simulink model "C705_FLATEARTH_sim"  (R2016a)
settings: Solver=ode23tb  StartTime=0.0  StopTime=t_sim  FixedStep=Ts  RelTol=1e-2
values from neighbouring files (symbols this model uses):
  att0 = [deg2rad(phi0) deg2rad(theta0) deg2rad(psi0)]    [C705_FLATEARTH_init2.m]
  boost = 30000    [C705_CFD_parameter.m]
  C = [-0.00159261761698 -0.0785492193562 0 0 0 0 0 0 -0.0394443854537 -0.0139411758211 0 0 ... (48 elements, 1x48)]    [C705CFDv2.mat]
  C3to4 = [1 -1 1;1 1 1;-1 1 1;-1 -1 1]    [C705_CFD_parameter.m]    (also in C705_FLATEARTH_init2.m)
  C4to3 = (1/4)*[1 1 -1 -1;-1 1 1 -1;1 1 1 1]    [C705_CFD_parameter.m]    (also in C705_FLATEARTH_init2.m)
  d_transisi = 2e3    (= 2000)    [C705_FLATEARTH_init2.m]
  dela_max = deg2rad(10)    [C705_FLATEARTH_init2.m]
  dele_max = deg2rad(10)    [C705_FLATEARTH_init2.m]
  delr_max = deg2rad(10)    [C705_FLATEARTH_init2.m]
  dmdt = -m_fuel/tmax    (= -0.04)    [C705_CFD_parameter.m]
  f_camera = 0.1    [C705_FLATEARTH_init2.m]
  fmax = (10/180)*pi    (= 0.174532925199)    [C705_CFD_parameter.m]    (also in C705_FLATEARTH_init2.m = deg2rad(10))
  k0 = 1    [C705_FLATEARTH_init2.m]
  Khdot = -1    [C705_FLATEARTH_init2.m]
  Ki_ay = -0.0024    [C705_FLATEARTH_init2.m]
  Ki_az = 0.0085    [C705_FLATEARTH_init2.m]
  Ki_psi = 4.1865e-07    [C705_FLATEARTH_init2.m]
  Ki_theta = 2.1878e-7    (= 2.1878e-07)    [C705_FLATEARTH_init2.m]
  Kiphi = 2e-7    (= 2e-07)    [C705_FLATEARTH_init2.m]
  Kp = -1.3248    [C705_FLATEARTH_init2.m]
  Kp_ay = -0.0135    [C705_FLATEARTH_init2.m]
  Kp_az = 0.0119    [C705_FLATEARTH_init2.m]
  Kp_h = 0.45    [C705_FLATEARTH_init2.m]
  Kp_psi = 1.7937    [C705_FLATEARTH_init2.m]
  Kp_theta = 1.7024    [C705_FLATEARTH_init2.m]
  Kphi = 1.8594    [C705_FLATEARTH_init2.m]
  Kq = 3.8200    (= 3.82)    [C705_FLATEARTH_init2.m]
  Kq_theta = -3.1594    [C705_FLATEARTH_init2.m]
  Kr = -10.1447    [C705_FLATEARTH_init2.m]
  Kr_psi = 8.6031    [C705_FLATEARTH_init2.m]
  Lref = 3.675    [C705_CFD_parameter.m]
  m_init = m_full-m_boost    (= 286)    [C705_CFD_parameter.m]
  N = 3    [C705_FLATEARTH_init2.m]
  p0 = [0,0,-h0]    [C705_FLATEARTH_init2.m]
  p1 = [6000,100,-200]    [C705_FLATEARTH_init2.m]
  p2 = [12000,300,-200]    [C705_FLATEARTH_init2.m]
  p3 = [18000,700,-200]    [C705_FLATEARTH_init2.m]
  pt = [24000,1000,0]    [C705_FLATEARTH_init2.m]
  Sref = 0.1711917    [C705_CFD_parameter.m]
  t_activate_del_a = 3    [C705_FLATEARTH_init2.m]
  t_activate_del_e = 5    [C705_FLATEARTH_init2.m]
  t_activate_del_r = 5    [C705_FLATEARTH_init2.m]
  tboost = 3    [C705_FLATEARTH_init2.m]
  TH = 3    [C705_FLATEARTH_init2.m]
  thrust = 910    [C705_CFD_parameter.m]
  Ts_ap = 1/Fs_ap    (= 0.005)    [C705_FLATEARTH_init2.m]
  Ts_guid = 1/Fs_guid    (= 0.005)    [C705_FLATEARTH_init2.m]
  tswitch = 0    [C705_FLATEARTH_init2.m]
  vb0 = [1e-3 0 0]    [C705_FLATEARTH_init2.m]
  wb0 = [0 0 0]    [C705_FLATEARTH_init2.m]
undefined symbols (not defined in the file or in its folder): DiscIntNeverNeededParam, F, GIr, GPr, K1r, K2r, Kda, Ki_h, Ki_p, Kp_p, Light, MIL
libraries: simulink x11, aerolibasang x4, aerolibguid x3, aerolibwind2 x3, aerolibutil x2, aerolibanim x1, aerolibactuator x1, aerolibtransform2 x1, aerolibatmos2 x1, aerolibgravity2 x1, aerolibbdyn x1, aerolibnav x1
(part 1 of 2)
settings Model: Creator=tommypra97  LastModifiedBy=LABSSAJ204
settings DataIOCC: LimitDataPoints=on  SaveFormat=StructureWithTime  SignalLoggingSaveFormat=ModelDataLogs  SaveTime=off
settings DebuggingCC: FcnCallInpInsideContextMsg=EnableAllAsWarning
settings HardwareCC: ProdBitPerPointer=32  ProdLargestAtomicFloat=None  ProdWordSize=32  ProdHWDeviceType=Specified
settings ModelReferenceCC: PropagateSignalLabelsOutOfModel=off
settings GRTTargetCC: CombineOutputUpdateFcns=off  GRTInterface=on

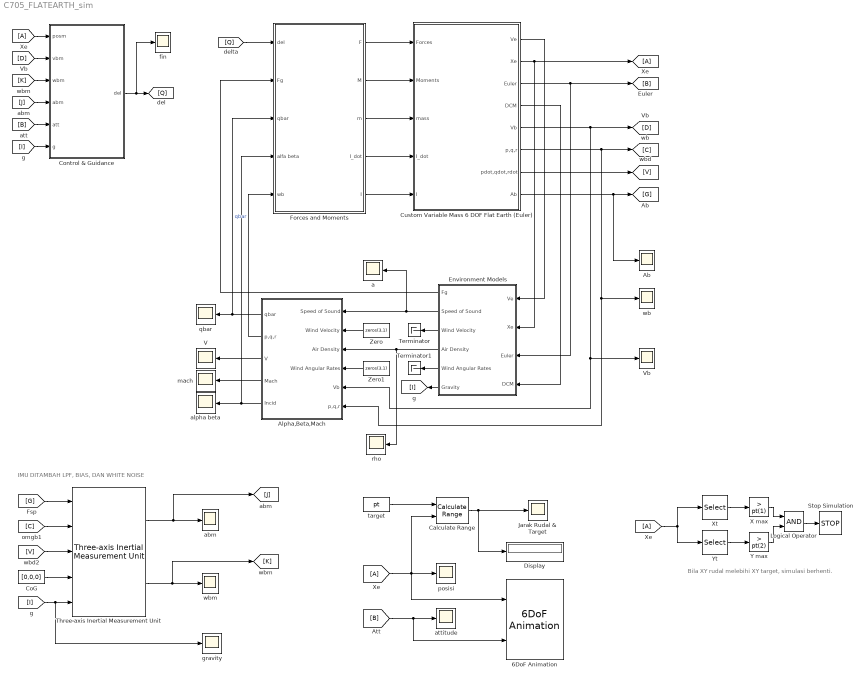
== system C705_FLATEARTH_sim ==
  note: Bila XY rudal melebihi XY target, simulasi berhenti.
  note: IMU DITAMBAH LPF, BIAS, DAN WHITE NOISE
  " Vb " : Scope
  " wb " : Scope
  6DoF Animation : aerolibanim/6DoF Animation  u1=[0 1 0 1 0 1]  u2=0.03  u3=7  u4=pt  u5=Fly alongside  u6=[-20 0 -7]  u7=20  u8=on
  "Ab " : Scope
  Alpha,Beta,Mach : Subsystem
  Calculate Range : aerolibguid/Calculate Range
  CoG : Constant  Value=[0,0,0]
  Control & Guidance : Subsystem
  Custom Variable Mass 6 DOF Flat Earth (Euler) : Subsystem
  Display : Display
  Environment Models : Subsystem
  Forces and Moments : Subsystem
  Jarak Rudal & Target : Scope
  Logical Operator : Logic  AllPortsSameDT=off  OutDataTypeStr=boolean
  Stop Simulation : Stop
  Terminator : Terminator
  Terminator1 : Terminator
  Three-axis Inertial Measurement Unit : aerolibnav/Three-axis Inertial Measurement Unit  units=Metric (MKS)  imu=[0 0 0]  dtype_a=on  w_a=wn_lpf  z_a=zeta_lpf  a_sf_cc=[1 0 0; 0 1 0; 0 0 1]  a_bias=acc_bias  a_sat="[-inf  -inf  -inf  inf inf inf]"  dtype_g=on  w_g=wn_lpf  z_g=zeta_lpf  g_sf_cc=[1 0 0; 0 1 0; 0 0 1]  g_bias=gyr_bias  g_sens=[0 0 0]  g_sat="[-inf  -inf  -inf  inf inf inf]"  i_rand=on  i_seeds=imu_noise_seed  i_pow=imu_noise_pwr  i_Ts=Ts_imu
  V : Scope
  X max : simulink/Logic and Bit Operations/Compare To Constant  relop=>  const=pt(1)  OutDataTypeStr=boolean  ZeroCross=off
  Xt : Selector  InputPortWidth=3  IndexOptions=Index vector (dialog)  Indices=1  OutputSizes=1
  Y max : simulink/Logic and Bit Operations/Compare To Constant  relop=>  const=pt(2)  OutDataTypeStr=boolean  ZeroCross=off
  Yt : Selector  InputPortWidth=3  IndexOptions=Index vector (dialog)  Indices=2  OutputSizes=1
  Zero : Constant  Value=zeros(3,1)
  Zero1 : Constant  Value=zeros(3,1)
  a : Scope
  "abm " : Scope
  alpha beta : Scope
  attitude : Scope
  "fin " : Scope
  gravity : Scope
  mach : Scope
  posisi : Scope
  qbar : Scope
  rho : Scope
  target : Constant  Value=pt
  "wbm " : Scope
  wires:
  Custom Variable Mass 6 DOF Flat Earth (Euler)/6(p,q,r) -> " wb "/1, Alpha,Beta,Mach/6(p,q,r), [C]
  Custom Variable Mass 6 DOF Flat Earth (Euler)/7(pdot,qdot,rdot) -> [V]
  Custom Variable Mass 6 DOF Flat Earth (Euler)/4(DCM) -> Environment Models/4(DCM)
  Custom Variable Mass 6 DOF Flat Earth (Euler)/3(Euler) -> [B], Environment Models/3(Euler)
  Environment Models/2(Speed of Sound) -> a/1, Alpha,Beta,Mach/1(Speed of Sound)
  Environment Models/4(Air Density) -> Alpha,Beta,Mach/3(Air Density), rho/1
  [A] -> Calculate Range/2, 6DoF Animation/1, posisi/1
  target/1 -> Calculate Range/1
  Alpha,Beta,Mach/4(Mach) -> mach/1
  Environment Models/1(Fg) -> Forces and Moments/2(Fg)
  Alpha,Beta,Mach/5(Incid) -> alpha beta/1, Forces and Moments/4(alfa beta)
  Environment Models/6(Gravity) -> [I]
  [G] -> Three-axis Inertial Measurement Unit/1
  [C] -> Three-axis Inertial Measurement Unit/2
  CoG/1 -> Three-axis Inertial Measurement Unit/4
  [I] -> Three-axis Inertial Measurement Unit/5, gravity/1
  [V] -> Three-axis Inertial Measurement Unit/3
  [A] -> Control & Guidance/1(posm)
  [D] -> Control & Guidance/2(vbm)
  [K] -> Control & Guidance/3(wbm)
  [J] -> Control & Guidance/4(abm)
  Custom Variable Mass 6 DOF Flat Earth (Euler)/8(Ab) -> "Ab "/1, [G]
  Alpha,Beta,Mach/1(qbar) -> qbar/1, Forces and Moments/3(qbar)  "qbar"
  Alpha,Beta,Mach/3(V) -> V/1
  Three-axis Inertial Measurement Unit/1 -> [J], "abm "/1
  Three-axis Inertial Measurement Unit/2 -> [K], "wbm "/1
  [B] -> Control & Guidance/5(att)
  Zero/1 -> Alpha,Beta,Mach/2(Wind Velocity)
  Zero1/1 -> Alpha,Beta,Mach/4(Wind Angular Rates)
  Environment Models/3(Wind Velocity) -> Terminator/1
  Environment Models/5(Wind Angular Rates) -> Terminator1/1
  [Q] -> Forces and Moments/1(del)
  Calculate Range/1 -> Display/1, Jarak Rudal & Target/1
  [I] -> Control & Guidance/6(g)
  Control & Guidance/1(del) -> "fin "/1, [Q]
  Alpha,Beta,Mach/2("p,q,r ") -> Forces and Moments/5(wb)
  Custom Variable Mass 6 DOF Flat Earth (Euler)/5(Vb) -> Alpha,Beta,Mach/5(Vb), " Vb "/1, [D]
  Forces and Moments/1(F) -> Custom Variable Mass 6 DOF Flat Earth (Euler)/1(Forces)
  Forces and Moments/2(M) -> Custom Variable Mass 6 DOF Flat Earth (Euler)/2(Moments)
  [B] -> attitude/1, 6DoF Animation/2
  Y max/1 -> Logical Operator/2
  X max/1 -> Logical Operator/1
  Logical Operator/1 -> Stop Simulation/1
  Xt/1 -> X max/1
  Yt/1 -> Y max/1
  Custom Variable Mass 6 DOF Flat Earth (Euler)/2(Xe) -> [A], Environment Models/2(Xe)
  Forces and Moments/5(I) -> Custom Variable Mass 6 DOF Flat Earth (Euler)/5(I)
  Forces and Moments/3(m) -> Custom Variable Mass 6 DOF Flat Earth (Euler)/3(mass)
  Forces and Moments/4(I_dot) -> Custom Variable Mass 6 DOF Flat Earth (Euler)/4(I_dot)
  Custom Variable Mass 6 DOF Flat Earth (Euler)/1(Ve) -> Environment Models/1(Ve)
  [A] -> Yt/1, Xt/1

== system C705_FLATEARTH_sim/Alpha,Beta,Mach ==
  Speed of Sound : Inport
  Wind Velocity : Inport  Port=2  PortDimensions=3
  Air Density : Inport  Port=3
  Wind Angular Rates : Inport  Port=4  PortDimensions=3
  Vb : Inport  Port=5  PortDimensions=3
  p,q,r : Inport  Port=6  PortDimensions=3
  Dynamic Pressure : aerolibasang/Dynamic Pressure
  "Incidence, Sideslip & Airspeed" : aerolibasang/Incidence, Sideslip, & Airspeed
  Mach Number : aerolibasang/Mach Number
  Mux : Mux  Inputs=2
  Sum : Sum  Inputs=|+-  SaturateOnIntegerOverflow=on  InputSameDT=on  OutDataTypeStr=Inherit: Same as first input
  Sum1 : Sum  Inputs=|++  SaturateOnIntegerOverflow=on  InputSameDT=on  OutDataTypeStr=Inherit: Same as first input
  qbar : Outport  InitialOutput=0
  "p,q,r " : Outport  Port=2
  V : Outport  Port=3
  Mach : Outport  Port=4
  Incid : Outport  Port=5
  wires:
  "Incidence, Sideslip & Airspeed"/3 -> V/1
  Dynamic Pressure/1 -> qbar/1
  Air Density/1 -> Dynamic Pressure/2
  Mach Number/1 -> Mach/1
  Sum/1 -> Dynamic Pressure/1, Mach Number/1, "Incidence, Sideslip & Airspeed"/1
  Vb/1 -> Sum/1
  Speed of Sound/1 -> Mach Number/2
  Wind Velocity/1 -> Sum/2
  "Incidence, Sideslip & Airspeed"/2 -> Mux/2  "Beta"
  Mux/1 -> Incid/1
  "Incidence, Sideslip & Airspeed"/1 -> Mux/1  "Alpha"
  p,q,r/1 -> Sum1/1
  Wind Angular Rates/1 -> Sum1/2
  Sum1/1 -> "p,q,r "/1

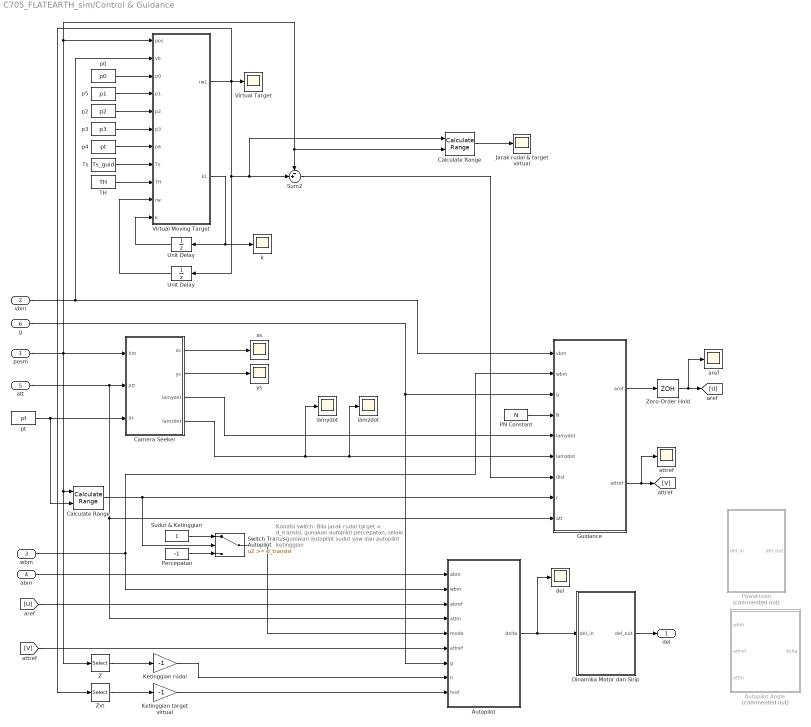
== system C705_FLATEARTH_sim/Control & Guidance ==
  note: Kondisi switch:
      | Bila jarak rudal-target < d_transisi,
      | gunakan autopilot percepatan,
      | selain itu, gunakan autopilot sudut yaw dan
      | autopilot ketinggian
  posm : Inport
  vbm : Inport  Port=2
  wbm : Inport  Port=3
  abm : Inport  Port=4
  att : Inport  Port=5
  g : Inport  Port=6
  Autopilot : Subsystem
  Autopilot Angle : Subsystem  Commented=on
  Calculate Range : aerolibguid/Calculate Range
  "Calculate Range " : aerolibguid/Calculate Range
  Camera Seeker : Subsystem
  Dinamika Motor dan Sirip : Subsystem
  Guidance : MATLAB Function  TreatAsAtomicUnit=on
  Jarak rudal & target virtual : Scope
  Ketinggian rudal : Gain  Gain=-1
  Ketinggian target virtual : Gain  Gain=-1
  PN Constant : Constant  Value=N
  Percepatan : Constant  Value=-1
  Pewaktuan : Subsystem  Commented=on
  Sudut & Ketinggian : Constant
  Sum2 : Sum  Inputs=-+|
  Switch Transisi Autopilot : Switch  Threshold=d_transisi
  TH : Constant  Value=TH
  Ts : Constant  Value=Ts_guid
  Unit Delay : UnitDelay  InitialCondition=k0  SampleTime=Ts_guid
  "Unit Delay " : UnitDelay  InitialCondition=p1  SampleTime=Ts_guid
  Virtual Moving Target : MATLAB Function  TreatAsAtomicUnit=on
  Virtual Target : Scope
  Z : Selector  InputPortWidth=3  IndexOptions=Index vector (dialog)  Indices=[3]  OutputSizes=1
  Zero-Order Hold : ZeroOrderHold  SampleTime=Ts_guid
  Zvt : Selector  InputPortWidth=3  IndexOptions=Index vector (dialog)  Indices=[3]  OutputSizes=1
  "aref " : Scope
  "attref " : Scope
  "del " : Scope
  k : Scope
  lamydot : Scope
  lamzdot : Scope
  p0 : Constant  Value=p0  VectorParams1D=off
  p2 : Constant  Value=p2
  p3 : Constant  Value=p3
  p4 : Constant  Value=pt
  p5 : Constant  Value=p1
  pt : Constant  Value=pt
  xs : Scope
  ys : Scope
  del : Outport
  wires:
  abm/1 -> Autopilot/1(abm)
  wbm/1 -> Autopilot/2(wbm), Guidance/2(wbm)
  g/1 -> Guidance/3(g), Autopilot/7(g)
  PN Constant/1 -> Guidance/4(N)
  Camera Seeker/1(xs) -> xs/1
  Camera Seeker/2(ys) -> ys/1
  Camera Seeker/3(lamydot) -> Guidance/5(lamydot)
  Camera Seeker/4(lamzdot) -> lamydot/1, lamzdot/1, Guidance/6(lamzdot)
  Zero-Order Hold/1 -> "aref "/1, [U]
  [U] -> Autopilot/3(abref)
  Guidance/1(aref) -> Zero-Order Hold/1
  p5/1 -> Virtual Moving Target/4(p1)
  p2/1 -> Virtual Moving Target/5(p2)
  p3/1 -> Virtual Moving Target/6(p3)
  p4/1 -> Virtual Moving Target/7(p4)
  vbm/1 -> Guidance/1(vbm), Virtual Moving Target/2(vb)
  Ts/1 -> Virtual Moving Target/8(Ts)
  "Unit Delay "/1 -> Virtual Moving Target/10(rw)
  Virtual Moving Target/2(k1) -> k/1, Unit Delay/1
  TH/1 -> Virtual Moving Target/9(TH)
  Unit Delay/1 -> Virtual Moving Target/11(k)
  p0/1 -> Virtual Moving Target/3(p0)
  Sum2/1 -> Guidance/7(dist)
  Guidance/2(attref) -> [V], "attref "/1
  posm/1 -> Calculate Range/1, Z/1, "Calculate Range "/2, Sum2/1, Virtual Moving Target/1(pos), Camera Seeker/1(Xm)
  pt/1 -> Calculate Range/2, Camera Seeker/3(Xt)
  "Calculate Range "/1 -> Jarak rudal & target virtual/1
  Calculate Range/1 -> Guidance/8(r), Switch Transisi Autopilot/2
  Autopilot/1(delta) -> "del "/1, Dinamika Motor dan Sirip/1(del_in)
  Dinamika Motor dan Sirip/1(del_out) -> del/1
  att/1 -> Guidance/9(att), Autopilot/4(attm), Camera Seeker/2(Att)
  Switch Transisi Autopilot/1 -> Autopilot/5(mode)
  Percepatan/1 -> Switch Transisi Autopilot/3
  Sudut & Ketinggian/1 -> Switch Transisi Autopilot/1
  [V] -> Autopilot/6(attref)
  Z/1 -> Ketinggian rudal/1
  Ketinggian rudal/1 -> Autopilot/8(h)
  Zvt/1 -> Ketinggian target virtual/1
  Ketinggian target virtual/1 -> Autopilot/9(href)
  Virtual Moving Target/1(rw1) -> Zvt/1, "Calculate Range "/1, Sum2/2, "Unit Delay "/1, Virtual Target/1

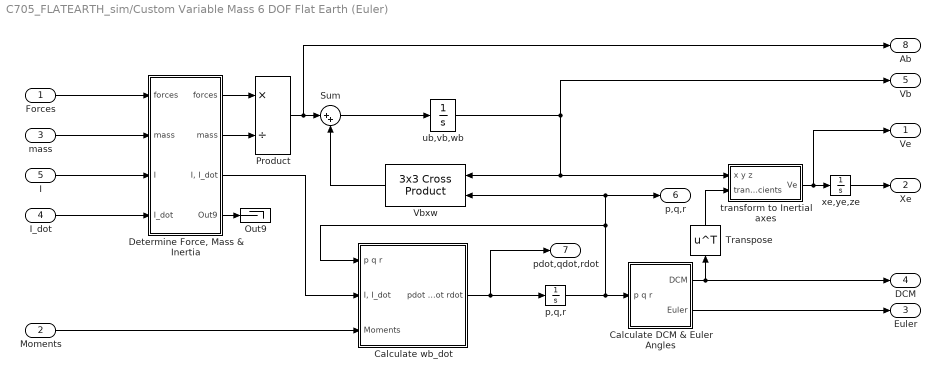
== system C705_FLATEARTH_sim/Custom Variable Mass 6 DOF Flat Earth (Euler) ==
  Forces : Inport  PortDimensions=3
  Moments : Inport  Port=2  PortDimensions=3
  mass : Inport  Port=3
  I_dot : Inport  Port=4  PortDimensions=[3 3]
  I : Inport  Port=5  PortDimensions=[3 3]
  Calculate DCM & Euler Angles : Subsystem
  "Calculate wb_dot " : Subsystem
  "Determine Force, Mass & Inertia " : Subsystem
  Out9 : Terminator
  Product : Product  Inputs=*/  SaturateOnIntegerOverflow=on  OutDataTypeStr=Inherit: Same as first input
  Sum : Sum  Inputs=|++  SaturateOnIntegerOverflow=on
  Transpose : Math  Operator=transpose  SaturateOnIntegerOverflow=on
  Vbxw : aerolibutil/3x3 Cross Product
  "p,q,r " : Integrator  InitialCondition=wb0
  transform to Inertial axes : Subsystem
  ub,vb,wb : Integrator  InitialCondition=vb0
  xe,ye,ze : Integrator  InitialCondition=p0
  Ve : Outport
  Xe : Outport  Port=2
  Euler : Outport  Port=3
  DCM : Outport  Port=4
  Vb : Outport  Port=5
  p,q,r : Outport  Port=6
  pdot,qdot,rdot : Outport  Port=7
  Ab : Outport  Port=8
  wires:
  Sum/1 -> ub,vb,wb/1
  "Determine Force, Mass & Inertia "/1("forces ") -> Product/1
  I_dot/1 -> "Determine Force, Mass & Inertia "/4(I_dot)
  "Calculate wb_dot "/1(pdot qdot rdot) -> pdot,qdot,rdot/1, "p,q,r "/1
  "Determine Force, Mass & Inertia "/4(Out9) -> Out9/1
  "Determine Force, Mass & Inertia "/2(mass) -> Product/2
  mass/1 -> "Determine Force, Mass & Inertia "/2("mass ")
  Transpose/1 -> transform to Inertial axes/2(transform coefficients)
  Calculate DCM & Euler Angles/1(DCM) -> DCM/1, Transpose/1
  ub,vb,wb/1 -> Vb/1, transform to Inertial axes/1(x y z), Vbxw/1
  transform to Inertial axes/1(Ve) -> Ve/1, xe,ye,ze/1
  Product/1 -> Ab/1, Sum/1
  Forces/1 -> "Determine Force, Mass & Inertia "/1(forces)
  I/1 -> "Determine Force, Mass & Inertia "/3(I)
  Moments/1 -> "Calculate wb_dot "/3(Moments)
  "p,q,r "/1 -> Calculate DCM & Euler Angles/1("p q r "), "Calculate wb_dot "/1(p q r), p,q,r/1, Vbxw/2
  Calculate DCM & Euler Angles/2(Euler) -> Euler/1
  Vbxw/1 -> Sum/2
  xe,ye,ze/1 -> Xe/1
  "Determine Force, Mass & Inertia "/3("I, I_dot ") -> "Calculate wb_dot "/2("I, I_dot")

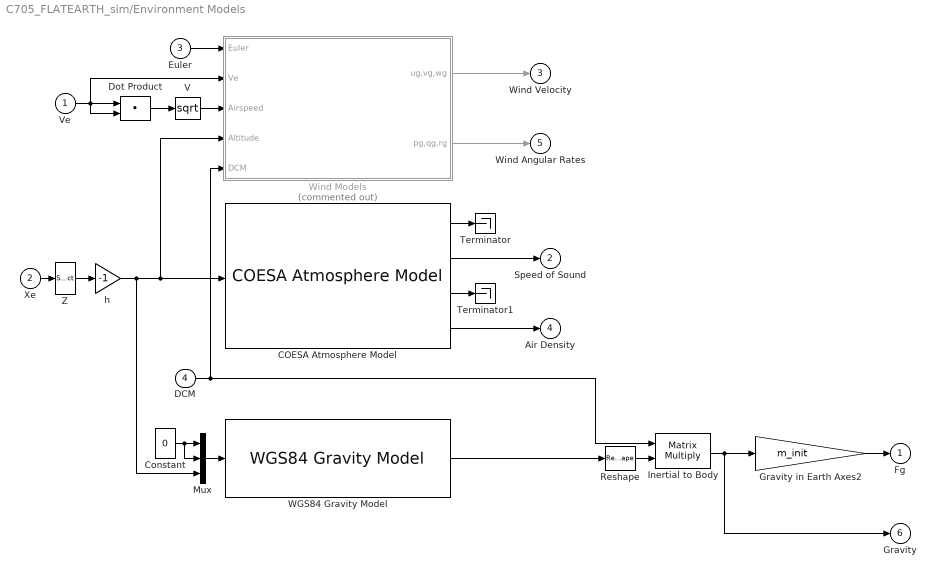
== system C705_FLATEARTH_sim/Environment Models ==
  Ve : Inport
  Xe : Inport  Port=2  PortDimensions=3
  Euler : Inport  Port=3
  DCM : Inport  Port=4
  COESA Atmosphere Model : aerolibatmos2/COESA Atmosphere Model  units=Metric (MKS)  spec=1976 COESA-extended U.S. Standard Atmosphere  model=Profile  profile_var=High temperature  profile_percent=10%  profile_alt=5 km (16404 ft)  envelope_var=High temperature  envelope_percent=1%  action=None
  Constant : Constant  Value=0
  Dot Product : DotProduct  SaturateOnIntegerOverflow=on  OutDataTypeStr=Inherit: Inherit via internal rule
  Gravity in Earth Axes2 : Gain  Gain=m_init  SaturateOnIntegerOverflow=on  OutDataTypeStr=Inherit: Same as input  ParamDataTypeStr=Inherit: Same as input
  Inertial to Body : Product  Multiplication=Matrix(*)  SaturateOnIntegerOverflow=on  InputSameDT=on  OutDataTypeStr=Inherit: Same as first input
  Mux : Mux  Inputs=3
  Reshape : Reshape
  Terminator : Terminator
  Terminator1 : Terminator
  V : Math  Operator=sqrt  SaturateOnIntegerOverflow=on
  "WGS84 Gravity Model " : aerolibgravity2/WGS84 Gravity Model   model=WGS84 Taylor Series  units=Metric (MKS)  no_atmos=on  precessing=on  jd_loc=off  month=October  day=10  year=2004  no_centrifugal=on  action=None
  Wind Models : Subsystem  Commented=on
  Z : Selector  InputPortWidth=3  IndexOptions=Index vector (dialog)  Indices=[3]  OutputSizes=1
  h : Gain  Gain=-1  SaturateOnIntegerOverflow=on  OutDataTypeStr=Inherit: Same as input  ParamDataTypeStr=Inherit: Same as input
  Fg : Outport  InitialOutput=0
  Speed of Sound : Outport  Port=2  InitialOutput=0
  Wind Velocity : Outport  Port=3  InitialOutput=0
  Air Density : Outport  Port=4  InitialOutput=0
  Wind Angular Rates : Outport  Port=5  InitialOutput=0
  Gravity : Outport  Port=6  InitialOutput=0
  wires:
  Reshape/1 -> Inertial to Body/2
  Euler/1 -> Wind Models/1(Euler)
  Ve/1 -> Wind Models/2(Ve), Dot Product/1, Dot Product/2
  Wind Models/1(ug,vg,wg) -> Wind Velocity/1
  Wind Models/2(pg,qg,rg) -> Wind Angular Rates/1
  Dot Product/1 -> V/1
  Z/1 -> h/1
  COESA Atmosphere Model/4 -> Air Density/1
  COESA Atmosphere Model/2 -> Speed of Sound/1
  COESA Atmosphere Model/3 -> Terminator1/1
  COESA Atmosphere Model/1 -> Terminator/1
  DCM/1 -> Wind Models/5(DCM), Inertial to Body/1
  V/1 -> Wind Models/3(Airspeed)
  "WGS84 Gravity Model "/1 -> Reshape/1
  Xe/1 -> Z/1
  Inertial to Body/1 -> Gravity/1, Gravity in Earth Axes2/1
  Gravity in Earth Axes2/1 -> Fg/1
  Mux/1 -> "WGS84 Gravity Model "/1
  Constant/1 -> Mux/2, Mux/1
  h/1 -> Mux/3, COESA Atmosphere Model/1, Wind Models/4(Altitude)

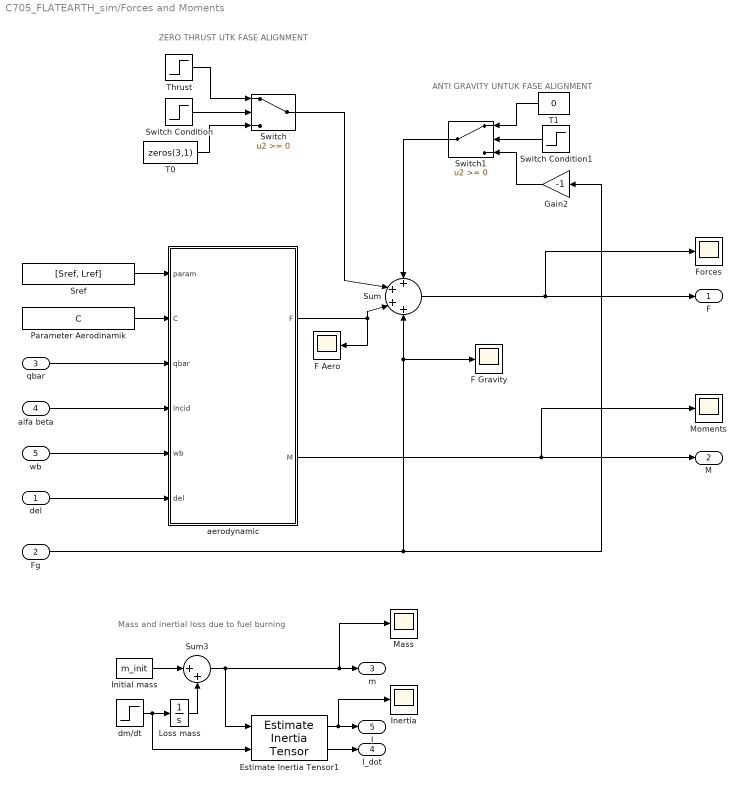
== system C705_FLATEARTH_sim/Forces and Moments ==
  note: ZERO THRUST UTK FASE ALIGNMENT
  note: ANTI GRAVITY UNTUK FASE ALIGNMENT
  note: Mass and inertial loss due to fuel burning
  del : Inport
  Fg : Inport  Port=2
  qbar : Inport  Port=3
  alfa beta : Inport  Port=4
  wb : Inport  Port=5
  " dm/dt " : Step  Time=tboost  Before=dmdt  After=0  SampleTime=0
  Estimate Inertia Tensor1 : aerolibbdyn/Estimate Inertia Tensor  fmass=m_init  emass=m_end  fI=I_init  eI=I_end
  F Aero : Scope
  F Gravity : Scope
  Forces : Scope
  Gain2 : Gain  Gain=-1
  "Inertia " : Scope
  Initial mass : Constant  Value=m_init
  Loss mass : Integrator
  Mass : Scope
  Moments : Scope
  Parameter Aerodinamik : Constant  Value=C  SampleTime=Ts_guid
  Sref : Constant  Value=[Sref, Lref]  SampleTime=Ts_guid
  Sum : Sum  Inputs=+|+|+|+  SaturateOnIntegerOverflow=on  InputSameDT=on  OutDataTypeStr=Inherit: Same as first input
  Sum3 : Sum  Inputs=|++  SaturateOnIntegerOverflow=on  InputSameDT=on  OutDataTypeStr=Inherit: Same as first input
  Switch : Switch
  Switch Condition : Step  Time=tswitch  Before=-1  SampleTime=0
  Switch Condition1 : Step  Time=tswitch  Before=-1  SampleTime=0
  Switch1 : Switch
  T0 : Constant  Value=zeros(3,1)  SampleTime=Ts_guid
  T1 : Constant  Value=0  SampleTime=Ts_guid
  Thrust : Step  Time=tswitch+tboost  Before=[boost 0 0]  After=[thrust 0 0]  SampleTime=0
  aerodynamic : MATLAB Function  TreatAsAtomicUnit=on
  F : Outport
  M : Outport  Port=2
  m : Outport  Port=3
  I_dot : Outport  Port=4
  I : Outport  Port=5
  wires:
  alfa beta/1 -> aerodynamic/4(incid)
  aerodynamic/1(F) -> Sum/3, F Aero/1
  qbar/1 -> aerodynamic/3(qbar)
  Sum/1 -> F/1, Forces/1
  Sref/1 -> aerodynamic/1(param)
  Parameter Aerodinamik/1 -> aerodynamic/2(C)
  aerodynamic/2(M) -> Moments/1, M/1
  del/1 -> aerodynamic/6(del)
  Switch Condition/1 -> Switch/2
  T0/1 -> Switch/3
  Thrust/1 -> Switch/1
  Switch Condition1/1 -> Switch1/2
  Gain2/1 -> Switch1/3
  T1/1 -> Switch1/1
  Switch1/1 -> Sum/1
  Switch/1 -> Sum/2
  wb/1 -> aerodynamic/5(wb)
  Fg/1 -> Sum/4, F Gravity/1, Gain2/1
  Estimate Inertia Tensor1/2 -> I_dot/1
  Estimate Inertia Tensor1/1 -> "Inertia "/1, I/1
  Initial mass/1 -> Sum3/1
  " dm/dt "/1 -> Estimate Inertia Tensor1/2, Loss mass/1
  Loss mass/1 -> Sum3/2
  Sum3/1 -> Estimate Inertia Tensor1/1, Mass/1, m/1

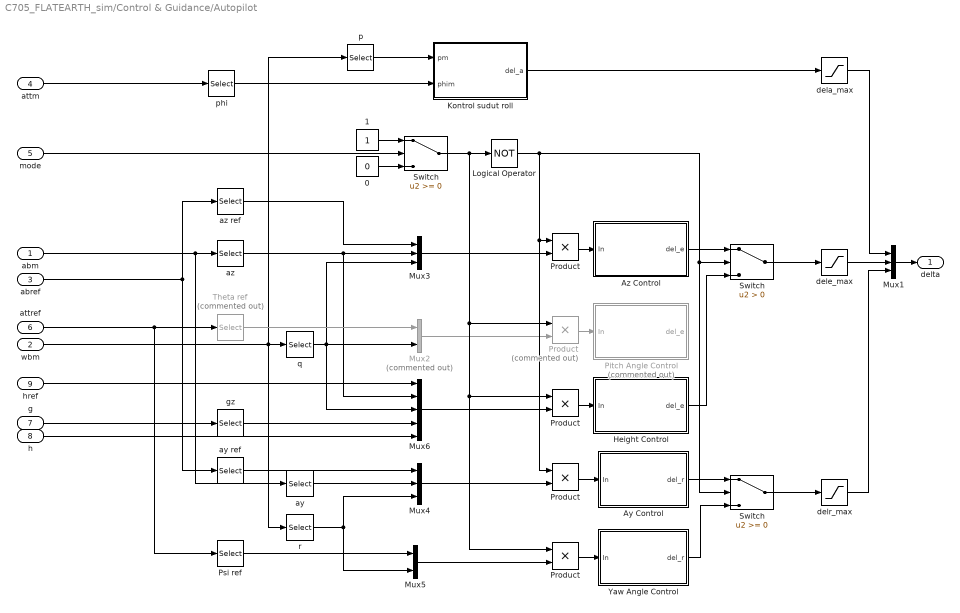
== system C705_FLATEARTH_sim/Control & Guidance/Autopilot ==
  abm : Inport
  wbm : Inport  Port=2
  abref : Inport  Port=3
  attm : Inport  Port=4
  mode : Inport  Port=5
  attref : Inport  Port=6
  g : Inport  Port=7
  h : Inport  Port=8
  href : Inport  Port=9
  " Product " : Product
  0 : Constant  Value=0
  1 : Constant
  Ay Control : Subsystem
  Az Control : Subsystem
  Height Control : Subsystem
  Kontrol sudut roll : Subsystem
  Logical Operator : Logic  Operator=NOT  AllPortsSameDT=off  OutDataTypeStr=boolean
  Mux1 : Mux  Inputs=3
  Mux2 : Mux  Commented=on  Inputs=2
  Mux3 : Mux  Inputs=3
  Mux4 : Mux  Inputs=3
  Mux5 : Mux  Inputs=2
  Mux6 : Mux  Inputs=5
  Pitch Angle Control : Subsystem  Commented=on
  Product : Product
  "Product " : Product  Commented=on
  "Product  " : Product
  "Product   " : Product
  Psi ref : Selector  InputPortWidth=3  IndexOptions=Index vector (dialog)  Indices=[3]  OutputSizes=1
  Switch : Switch
  "Switch " : Switch  Criteria=u2 > Threshold
  "Switch  " : Switch
  Theta ref : Selector  Commented=on  InputPortWidth=3  IndexOptions=Index vector (dialog)  Indices=2  OutputSizes=1
  Yaw Angle Control : Subsystem
  ay : Selector  InputPortWidth=3  IndexOptions=Index vector (dialog)  Indices=[2]  OutputSizes=1
  ay ref : Selector  InputPortWidth=3  IndexOptions=Index vector (dialog)  Indices=[2]  OutputSizes=1
  "az " : Selector  InputPortWidth=3  IndexOptions=Index vector (dialog)  Indices=[3]  OutputSizes=1
  az ref : Selector  InputPortWidth=3  IndexOptions=Index vector (dialog)  Indices=[3]  OutputSizes=1
  dela_max : Saturate  UpperLimit=dela_max  LowerLimit=-dela_max
  dele_max : Saturate  UpperLimit=dele_max  LowerLimit=-dele_max
  delr_max : Saturate  UpperLimit=delr_max  LowerLimit=-delr_max
  gz : Selector  InputPortWidth=3  IndexOptions=Index vector (dialog)  Indices=[3]  OutputSizes=1
  p : Selector  InputPortWidth=3  IndexOptions=Index vector (dialog)  Indices=[1]  OutputSizes=1
  phi : Selector  InputPortWidth=3  IndexOptions=Index vector (dialog)  Indices=[1]  OutputSizes=1
  q : Selector  InputPortWidth=3  IndexOptions=Index vector (dialog)  Indices=[2]  OutputSizes=1
  r : Selector  InputPortWidth=3  IndexOptions=Index vector (dialog)  Indices=[3]  OutputSizes=1
  delta : Outport
  wires:
  abref/1 -> az ref/1, ay ref/1
  wbm/1 -> q/1, p/1, r/1
  abm/1 -> "az "/1, ay/1
  p/1 -> Kontrol sudut roll/1(pm)
  Kontrol sudut roll/1(del_a) -> dela_max/1
  r/1 -> Mux5/2, Mux4/3
  az ref/1 -> Mux3/1
  attm/1 -> phi/1
  phi/1 -> Kontrol sudut roll/2(phim)
  dele_max/1 -> Mux1/2
  dela_max/1 -> Mux1/1
  delr_max/1 -> Mux1/3
  Mux1/1 -> delta/1
  q/1 -> Mux6/3, Mux3/3, Mux2/2
  mode/1 -> Switch/2
  0/1 -> Switch/3
  "az "/1 -> Mux6/2, Mux3/2
  Mux3/1 -> Product/2
  1/1 -> Switch/1
  Theta ref/1 -> Mux2/1
  Mux2/1 -> "Product "/2
  Switch/1 -> " Product "/1, "Product   "/1, "Product "/1, Logical Operator/1
  "Product "/1 -> Pitch Angle Control/1(In)
  Logical Operator/1 -> "Switch "/2, "Switch  "/2, "Product  "/1, Product/1
  Product/1 -> Az Control/1(In)
  ay ref/1 -> Mux4/1
  ay/1 -> Mux4/2
  Psi ref/1 -> Mux5/1
  Mux4/1 -> "Product  "/2
  Mux5/1 -> "Product   "/2
  "Product   "/1 -> Yaw Angle Control/1(In)
  "Product  "/1 -> Ay Control/1(In)
  Az Control/1(del_e) -> "Switch "/1
  Height Control/1(del_e) -> "Switch "/3
  "Switch "/1 -> dele_max/1
  Ay Control/1(del_r) -> "Switch  "/1
  Yaw Angle Control/1(del_r) -> "Switch  "/3
  "Switch  "/1 -> delr_max/1
  attref/1 -> Psi ref/1, Theta ref/1
  g/1 -> gz/1
  gz/1 -> Mux6/4
  " Product "/1 -> Height Control/1(In)
  Mux6/1 -> " Product "/2
  href/1 -> Mux6/1
  h/1 -> Mux6/5

== system C705_FLATEARTH_sim/Control & Guidance/Autopilot Angle ==
  wbm : Inport
  attref : Inport  Port=2
  attm : Inport  Port=3
  "Incidence, Sideslip & Airspeed" : aerolibasang/Incidence, Sideslip, & Airspeed  Commented=on
  Mux1 : Mux  Inputs=3
  Pitch Angle Control : Subsystem
  Psi ref : Selector  InputPortWidth=3  IndexOptions=Index vector (dialog)  Indices=[3]  OutputSizes=1
  Theta ref : Selector  InputPortWidth=3  IndexOptions=Index vector (dialog)  Indices=2  OutputSizes=1
  Yaw Angle Control : Subsystem
  p : Selector  InputPortWidth=3  IndexOptions=Index vector (dialog)  Indices=[1]  OutputSizes=1
  phi : Selector  InputPortWidth=3  IndexOptions=Index vector (dialog)  Indices=[1]  OutputSizes=1
  q : Selector  InputPortWidth=3  IndexOptions=Index vector (dialog)  Indices=[2]  OutputSizes=1
  r : Selector  InputPortWidth=3  IndexOptions=Index vector (dialog)  Indices=[3]  OutputSizes=1
  roll control : Subsystem
  delta : Outport
  wires:
  attref/1 -> Theta ref/1, Psi ref/1
  wbm/1 -> q/1, p/1, r/1
  p/1 -> roll control/1(pm)
  r/1 -> Yaw Angle Control/2("r ")
  q/1 -> Pitch Angle Control/2(q)
  Theta ref/1 -> Pitch Angle Control/1(Theta ref)
  Psi ref/1 -> Yaw Angle Control/1(Psi ref)
  Pitch Angle Control/1(del_e) -> Mux1/2
  roll control/1(del_a) -> Mux1/1
  Yaw Angle Control/1(del_r) -> Mux1/3
  Mux1/1 -> delta/1
  attm/1 -> phi/1
  phi/1 -> roll control/2(phim)

== system C705_FLATEARTH_sim/Control & Guidance/Camera Seeker ==
  Xm : Inport
  Att : Inport  Port=2
  Xt : Inport  Port=3
  Derivative : Derivative
  "Derivative " : Derivative
  Screen Camera : MATLAB Function  TreatAsAtomicUnit=on
  camera focus : Constant  Value=f_camera
  lamy : Scope
  lamz : Scope
  limit : Saturate  UpperLimit=pi  LowerLimit=-pi  LinearizeAsGain=off  ZeroCross=off
  limit1 : Saturate  UpperLimit=pi  LowerLimit=-pi  LinearizeAsGain=off  ZeroCross=off
  xs : Outport
  ys : Outport  Port=2
  lamydot : Outport  Port=3
  lamzdot : Outport  Port=4
  wires:
  Screen Camera/2(ys) -> ys/1
  Screen Camera/1(xs) -> xs/1
  Att/1 -> Screen Camera/2(att)
  Xm/1 -> Screen Camera/1(xm)
  Xt/1 -> Screen Camera/3(xt)
  camera focus/1 -> Screen Camera/4(f)
  Screen Camera/3(lamy) -> lamy/1, Derivative/1
  Screen Camera/4(lamz) -> lamz/1, "Derivative "/1
  "Derivative "/1 -> limit1/1
  Derivative/1 -> limit/1
  limit1/1 -> lamzdot/1
  limit/1 -> lamydot/1

== system C705_FLATEARTH_sim/Control & Guidance/Dinamika Motor dan Sirip ==
  del_in : Inport
  Act2Aero : Gain  Gain=C4to3  Multiplication=Matrix(K*u)  SaturateOnIntegerOverflow=on  OutDataTypeStr=Inherit: Same as input  ParamDataTypeStr=Inherit: Same as input
  Aero2Act : Gain  Gain=C3to4  Multiplication=Matrix(K*u)  SaturateOnIntegerOverflow=on  OutDataTypeStr=Inherit: Same as input  ParamDataTypeStr=Inherit: Same as input
  Nonlinear Second-Order Actuator : aerolibactuator/Nonlinear Second-Order Actuator  wn_fin=wn_act  z_fin=zeta_act  fin_max=[fmax fmax fmax fmax]  fin_min=-[fmax fmax fmax fmax]  fin_maxrate=inf  fin_act_0=0  fin_act_vel=0
  Scope1 : Scope
  Scope3 : Scope
  del_out : Outport
  wires:
  Act2Aero/1 -> del_out/1
  del_in/1 -> Aero2Act/1
  Aero2Act/1 -> Nonlinear Second-Order Actuator/1, Scope1/1
  Nonlinear Second-Order Actuator/1 -> Scope3/1, Act2Aero/1

== system C705_FLATEARTH_sim/Control & Guidance/Pewaktuan ==
  del_in : Inport
  Demux1 : Demux  Outputs=3
  Mux3 : Mux  Inputs=3
  Switch Condition : Step  Time=t_activate_del_a  Before=-1  SampleTime=0
  Switch Condition1 : Step  Time=t_activate_del_r  Before=-1  SampleTime=0
  Switch Condition2 : Step  Time=t_activate_del_e  Before=-1  SampleTime=0
  Switch del_e : Switch
  Switch del_r : Switch
  Swith del_a : Switch
  Zero : Constant  Value=0  SampleTime=Ts_guid
  Zero(2) : Constant  Value=0  SampleTime=Ts_guid
  Zero(2)1 : Constant  Value=0  SampleTime=Ts_guid
  del_out : Outport
  wires:
  Switch Condition/1 -> Swith del_a/2
  Zero/1 -> Swith del_a/3
  Demux1/1 -> Swith del_a/1
  Switch Condition1/1 -> Switch del_r/2
  Zero(2)/1 -> Switch del_r/3
  Demux1/3 -> Switch del_r/1
  Switch Condition2/1 -> Switch del_e/2
  Zero(2)1/1 -> Switch del_e/3
  Demux1/2 -> Switch del_e/1
  del_in/1 -> Demux1/1
  Switch del_e/1 -> Mux3/2
  Swith del_a/1 -> Mux3/1
  Switch del_r/1 -> Mux3/3
  Mux3/1 -> del_out/1

== system C705_FLATEARTH_sim/Custom Variable Mass 6 DOF Flat Earth (Euler)/Calculate DCM & Euler Angles ==
  "p q r " : Inport
  Rotation Angles to Direction Cosine Matrix : aerolibtransform2/Rotation Angles to Direction Cosine Matrix  rotationOrder=ZYX
  Selector : Selector  InputPortWidth=3  IndexOptions=Index vector (dialog)  Indices=[3 2 1]  OutputSizes=1
  phi theta psi : Integrator  InitialCondition=att0
  "phidot thetadot psidot " : Subsystem
  DCM : Outport
  Euler : Outport  Port=2
  wires:
  Selector/1 -> Rotation Angles to Direction Cosine Matrix/1
  phi theta psi/1 -> "phidot thetadot psidot "/2(phi theta psi), Euler/1, Selector/1
  "phidot thetadot psidot "/1(phidot thetadot psi) -> phi theta psi/1
  "p q r "/1 -> "phidot thetadot psidot "/1(p q r)
  Rotation Angles to Direction Cosine Matrix/1 -> DCM/1

== system C705_FLATEARTH_sim/Custom Variable Mass 6 DOF Flat Earth (Euler)/Calculate wb_dot  ==
  p q r : Inport
  "I, I_dot" : Inport  Port=2
  Moments : Inport  Port=3
  I*wb : Subsystem
  Idot*wb : Subsystem
  Product2 : Product  Inputs=*/  Multiplication=Matrix(*)  SaturateOnIntegerOverflow=on  OutDataTypeStr=Inherit: Same as first input
  Reshape : Reshape
  Reshape1 : Reshape  OutputDimensionality=Row vector (2-D)
  Selector : Selector  NumberOfDimensions=2  InputPortWidth=2  IndexOptions=Index vector (dialog),Select all  Indices=1:3,-1  OutputSizes=1
  Selector1 : Selector  NumberOfDimensions=2  InputPortWidth=2  IndexOptions=Index vector (dialog),Select all  Indices=4:6,-1  OutputSizes=1
  Selector2 : Selector  NumberOfDimensions=2  InputPortWidth=2  IndexOptions=Index vector (dialog),Select all  Indices=1:3,-1  OutputSizes=1
  Sum2 : Sum  Inputs=+--  SaturateOnIntegerOverflow=on
  wx(Iw) : aerolibutil/3x3 Cross Product
  pdot qdot rdot : Outport
  wires:
  Reshape1/1 -> Product2/1
  I*wb/1(I * w) -> wx(Iw)/2
  wx(Iw)/1 -> Sum2/3
  Selector1/1 -> Idot*wb/1(I_dot)
  Moments/1 -> Sum2/1
  Sum2/1 -> Reshape1/1
  Product2/1 -> Reshape/1
  p q r/1 -> I*wb/1(p q r), Idot*wb/2(p q r), wx(Iw)/1
  "I, I_dot"/1 -> Selector2/1, Selector/1, Selector1/1
  Selector2/1 -> Product2/2
  Reshape/1 -> pdot qdot rdot/1
  Idot*wb/1(Id * w) -> Sum2/2
  Selector/1 -> I*wb/2(Inertia)

== system C705_FLATEARTH_sim/Custom Variable Mass 6 DOF Flat Earth (Euler)/Determine Force, Mass & Inertia  ==
  forces : Inport
  "mass " : Inport  Port=2
  I : Inport  Port=3
  I_dot : Inport  Port=4
  Ground : Ground
  Matrix Concatenation : Concatenate  Mode=Multidimensional array
  "forces " : Outport
  mass : Outport  Port=2
  "I, I_dot " : Outport  Port=3
  Out9 : Outport  Port=4
  wires:
  Ground/1 -> Out9/1
  I/1 -> Matrix Concatenation/1
  "mass "/1 -> mass/1
  Matrix Concatenation/1 -> "I, I_dot "/1
  I_dot/1 -> Matrix Concatenation/2
  forces/1 -> "forces "/1

== system C705_FLATEARTH_sim/Custom Variable Mass 6 DOF Flat Earth (Euler)/transform to Inertial axes ==
  x y z : Inport
  transform coefficients : Inport  Port=2
  Product : Product  Multiplication=Matrix(*)  SaturateOnIntegerOverflow=on  InputSameDT=on  OutDataTypeStr=Inherit: Same as first input
  Reshape1 : Reshape  OutputDimensionality=Column vector (2-D)
  Reshape2 : Reshape
  Ve : Outport
  wires:
  Reshape2/1 -> Ve/1
  Reshape1/1 -> Product/2
  x y z/1 -> Reshape1/1
  transform coefficients/1 -> Product/1
  Product/1 -> Reshape2/1

== system C705_FLATEARTH_sim/Environment Models/Wind Models ==
  Euler : Inport
  Ve : Inport  Port=2
  Airspeed : Inport  Port=3
  Altitude : Inport  Port=4
  DCM : Inport  Port=5
  Discrete Wind Gust Model - On : aerolibwind2/Discrete Wind Gust Model  units=Metric (MKS)  Gx=on  Gy=on  Gz=on  t_0=20  d_m=[120 120 80]  v_m=[3.5 3.0 3.0]
  Dryden Wind Turbulence Model (Continuous (+q -r)) : aerolibwind2/Dryden Wind Turbulence Model  (Continuous (+q -r))  units=Metric (MKS)  spec=MIL-F-8785C  model=Continuous Dryden (+q -r)  W20=5  Wdeg=0  TurbProb=10^-2 - Light  L_high=533.4  Wingspan=4  ts=0.1  Seed=[23341 23342 23343 23344]  T_on=on
  Sum : Sum  Inputs=+++  SaturateOnIntegerOverflow=on  InputSameDT=on  OutDataTypeStr=Inherit: Same as first input
  Terminator : Terminator
  Terminator1 : Terminator
  Wind Shear Model : aerolibwind2/Wind Shear Model  units=Metric (MKS)  phase=Category C - Terminal Flight Phase  W_20=1  Wdeg=0
  ug,vg,wg : Outport
  pg,qg,rg : Outport  Port=2
  wires:
  Euler/1 -> Terminator1/1
  Ve/1 -> Terminator/1
  Wind Shear Model/1 -> Sum/1
  Dryden Wind Turbulence Model (Continuous (+q -r))/1 -> Sum/2
  Discrete Wind Gust Model - On/1 -> Sum/3
  Sum/1 -> ug,vg,wg/1
  DCM/1 -> Dryden Wind Turbulence Model (Continuous (+q -r))/3, Wind Shear Model/2
  Airspeed/1 -> Dryden Wind Turbulence Model (Continuous (+q -r))/2, Discrete Wind Gust Model - On/1
  Dryden Wind Turbulence Model (Continuous (+q -r))/2 -> pg,qg,rg/1
  Altitude/1 -> Dryden Wind Turbulence Model (Continuous (+q -r))/1, Wind Shear Model/1

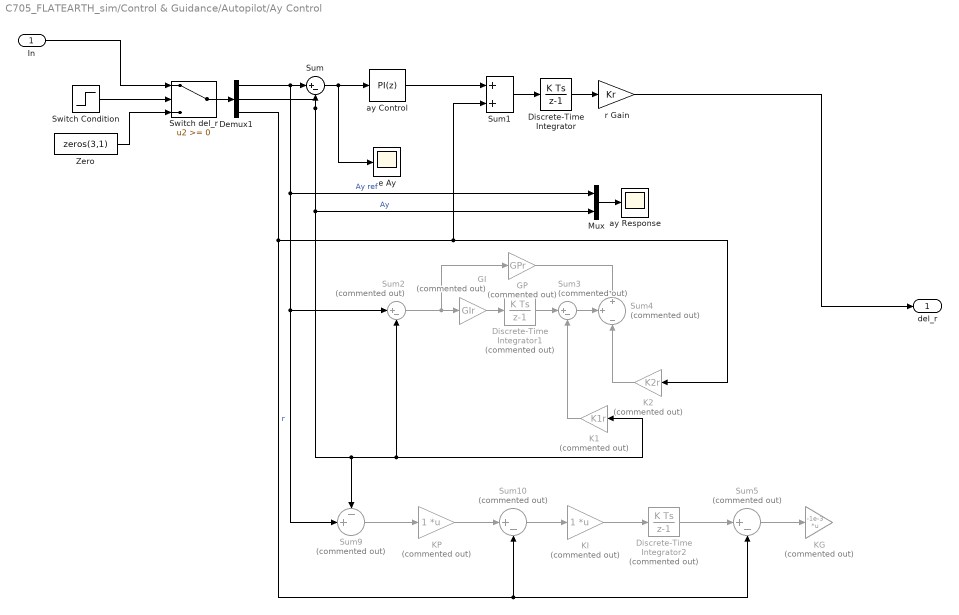
== system C705_FLATEARTH_sim/Control & Guidance/Autopilot/Ay Control ==
  In : Inport
  Demux1 : Demux  Outputs=3
  Discrete-Time Integrator : DiscreteIntegrator  InitialConditionSetting=State (most efficient)  SampleTime=Ts_ap  ICPrevOutput=DiscIntNeverNeededParam  ICPrevScaledInput=DiscIntNeverNeededParam
  Discrete-Time Integrator1 : DiscreteIntegrator  Commented=on  SampleTime=Ts_ap  ICPrevOutput=DiscIntNeverNeededParam  ICPrevScaledInput=DiscIntNeverNeededParam
  Discrete-Time Integrator2 : DiscreteIntegrator  Commented=on  SampleTime=Ts_ap  ICPrevOutput=DiscIntNeverNeededParam  ICPrevScaledInput=DiscIntNeverNeededParam
  GI : Gain  Commented=on  Gain=GIr
  GP : Gain  Commented=on  Gain=GPr
  K1 : Gain  Commented=on  Gain=K1r
  K2 : Gain  Commented=on  Gain=K2r
  KG : Gain  Commented=on  Gain=-1e-3  Multiplication=Matrix(K*u)  SaturateOnIntegerOverflow=on  OutDataTypeStr=Inherit: Same as input  ParamDataTypeStr=Inherit: Same as input
  KI : Gain  Commented=on  Multiplication=Matrix(K*u)  SaturateOnIntegerOverflow=on  OutDataTypeStr=Inherit: Same as input  ParamDataTypeStr=Inherit: Same as input
  KP : Gain  Commented=on  Multiplication=Matrix(K*u)  SaturateOnIntegerOverflow=on  OutDataTypeStr=Inherit: Same as input  ParamDataTypeStr=Inherit: Same as input
  Mux : Mux  Inputs=2
  Sum : Sum  Inputs=|+-  SaturateOnIntegerOverflow=on
  Sum1 : Sum  SaturateOnIntegerOverflow=on
  Sum10 : Sum  Commented=on  Inputs=|+-  SaturateOnIntegerOverflow=on  InputSameDT=on  OutDataTypeStr=Inherit: Same as first input
  Sum2 : Sum  Commented=on  Inputs=|+-
  Sum3 : Sum  Commented=on  Inputs=|+-
  Sum4 : Sum  Commented=on  Inputs=+|+|-
  Sum5 : Sum  Commented=on  Inputs=|+-  SaturateOnIntegerOverflow=on  InputSameDT=on  OutDataTypeStr=Inherit: Same as first input
  Sum9 : Sum  Commented=on  Inputs=-+|  SaturateOnIntegerOverflow=on  InputSameDT=on  OutDataTypeStr=Inherit: Same as first input
  Switch Condition : Step  Time=t_activate_del_r  Before=-1  SampleTime=0
  Switch del_r : Switch
  Zero : Constant  Value=zeros(3,1)  SampleTime=Ts_guid
  ay Control : simulink/Continuous/PID Controller  Controller=PI  TimeDomain=Discrete-time  SampleTime=Ts_ap  IntegratorMethod=Trapezoidal  FilterMethod=Forward Euler  Form=Parallel  UseFilter=on  ControllerParametersSource=internal  P=Kp_ay  I=Ki_ay  D=0  N=12  InitialConditionSource=internal  InitialConditionForIntegrator=0  InitialConditionForFilter=0  ExternalReset=none  LimitOutput=off  UpperSaturationLimit=inf  LowerSaturationLimit=-inf  LinearizeAsGain=off  AntiWindupMode=none  Kb=1  TrackingMode=off  Kt=1  PParamMin=[]  PParamMax=[]  IParamMin=[]  IParamMax=[]  DParamMin=[]  DParamMax=[]  NParamMin=[]  NParamMax=[]  KbParamMin=[]  KbParamMax=[]  KtParamMin=[]  KtParamMax=[]  POutMin=[]  POutMax=[]  IOutMin=[]  IOutMax=[]  DOutMin=[]  DOutMax=[]  NOutMin=[]  NOutMax=[]  KbOutMin=[]  KbOutMax=[]  KtOutMin=[]  KtOutMax=[]  IntegratorOutMin=[]  IntegratorOutMax=[]  FilterOutMin=[]  FilterOutMax=[]  SumOutMin=[]  SumOutMax=[]  SumI1OutMin=[]  SumI1OutMax=[]  SumI2OutMin=[]  SumI2OutMax=[]  SumI3OutMin=[]  SumI3OutMax=[]  SumDOutMin=[]  SumDOutMax=[]  SaturationOutMin=[]  SaturationOutMax=[]  IntegratorContinuousStateAttributes=''  IntegratorStateMustResolveToSignalObject=off  IntegratorRTWStateStorageClass=Auto  FilterContinuousStateAttributes=''  FilterStateMustResolveToSignalObject=off  FilterRTWStateStorageClass=Auto  DifferentiatorICPrevScaledInput=0  DifferentiatorOutMin=[]  DifferentiatorOutMax=[]
  ay Response : Scope
  e Ay : Scope
  r Gain : Gain  Gain=Kr
  del_r : Outport
  wires:
  Sum/1 -> e Ay/1, ay Control/1
  ay Control/1 -> Sum1/1
  Sum1/1 -> Discrete-Time Integrator/1
  Sum2/1 -> GP/1, GI/1
  GI/1 -> Discrete-Time Integrator1/1
  Discrete-Time Integrator1/1 -> Sum3/1
  Sum3/1 -> Sum4/2
  GP/1 -> Sum4/1
  K1/1 -> Sum3/2
  K2/1 -> Sum4/3
  KP/1 -> Sum10/1
  Sum10/1 -> KI/1
  Demux1/1 -> Sum9/2, Sum2/1, Mux/1, Sum/1  "Ay ref"
  Demux1/3 -> Sum1/2, K2/1, Sum10/2, Sum5/2  "r"
  Demux1/2 -> Mux/2, Sum9/1, Sum2/2, K1/1, Sum/2  "Ay"
  KI/1 -> Discrete-Time Integrator2/1
  Discrete-Time Integrator2/1 -> Sum5/1
  Sum5/1 -> KG/1
  Sum9/1 -> KP/1
  Discrete-Time Integrator/1 -> r Gain/1
  r Gain/1 -> del_r/1
  Mux/1 -> ay Response/1
  Switch Condition/1 -> Switch del_r/2
  Zero/1 -> Switch del_r/3
  In/1 -> Switch del_r/1
  Switch del_r/1 -> Demux1/1

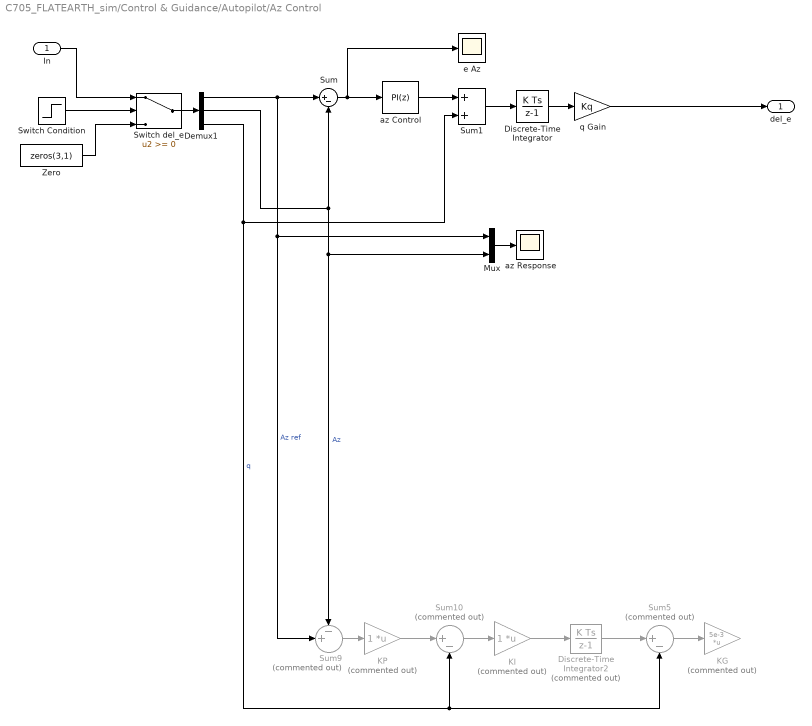
== system C705_FLATEARTH_sim/Control & Guidance/Autopilot/Az Control ==
  In : Inport
  Demux1 : Demux  Outputs=3
  Discrete-Time Integrator : DiscreteIntegrator  InitialConditionSetting=State (most efficient)  SampleTime=Ts_ap  ICPrevOutput=DiscIntNeverNeededParam  ICPrevScaledInput=DiscIntNeverNeededParam
  Discrete-Time Integrator2 : DiscreteIntegrator  Commented=on  SampleTime=Ts_ap  ICPrevOutput=DiscIntNeverNeededParam  ICPrevScaledInput=DiscIntNeverNeededParam
  KG : Gain  Commented=on  Gain=5e-3  Multiplication=Matrix(K*u)  SaturateOnIntegerOverflow=on  OutDataTypeStr=Inherit: Same as input  ParamDataTypeStr=Inherit: Same as input
  KI : Gain  Commented=on  Multiplication=Matrix(K*u)  SaturateOnIntegerOverflow=on  OutDataTypeStr=Inherit: Same as input  ParamDataTypeStr=Inherit: Same as input
  KP : Gain  Commented=on  Multiplication=Matrix(K*u)  SaturateOnIntegerOverflow=on  OutDataTypeStr=Inherit: Same as input  ParamDataTypeStr=Inherit: Same as input
  Mux : Mux  Inputs=2
  Sum : Sum  Inputs=|+-  SaturateOnIntegerOverflow=on
  Sum1 : Sum  SaturateOnIntegerOverflow=on
  Sum10 : Sum  Commented=on  Inputs=|+-  SaturateOnIntegerOverflow=on  InputSameDT=on  OutDataTypeStr=Inherit: Same as first input
  Sum5 : Sum  Commented=on  Inputs=|+-  SaturateOnIntegerOverflow=on  InputSameDT=on  OutDataTypeStr=Inherit: Same as first input
  Sum9 : Sum  Commented=on  Inputs=-+|  SaturateOnIntegerOverflow=on  InputSameDT=on  OutDataTypeStr=Inherit: Same as first input
  Switch Condition : Step  Time=t_activate_del_e  Before=-1  SampleTime=0
  Switch del_e : Switch
  Zero : Constant  Value=zeros(3,1)  SampleTime=Ts_guid
  az Control : simulink/Continuous/PID Controller  Controller=PI  TimeDomain=Discrete-time  SampleTime=Ts_ap  IntegratorMethod=Trapezoidal  FilterMethod=Forward Euler  Form=Parallel  UseFilter=on  ControllerParametersSource=internal  P=Kp_az  I=Ki_az  D=0  N=12  InitialConditionSource=internal  InitialConditionForIntegrator=0  InitialConditionForFilter=0  ExternalReset=none  LimitOutput=off  UpperSaturationLimit=inf  LowerSaturationLimit=-inf  LinearizeAsGain=off  AntiWindupMode=none  Kb=1  TrackingMode=off  Kt=1  PParamMin=[]  PParamMax=[]  IParamMin=[]  IParamMax=[]  DParamMin=[]  DParamMax=[]  NParamMin=[]  NParamMax=[]  KbParamMin=[]  KbParamMax=[]  KtParamMin=[]  KtParamMax=[]  POutMin=[]  POutMax=[]  IOutMin=[]  IOutMax=[]  DOutMin=[]  DOutMax=[]  NOutMin=[]  NOutMax=[]  KbOutMin=[]  KbOutMax=[]  KtOutMin=[]  KtOutMax=[]  IntegratorOutMin=[]  IntegratorOutMax=[]  FilterOutMin=[]  FilterOutMax=[]  SumOutMin=[]  SumOutMax=[]  SumI1OutMin=[]  SumI1OutMax=[]  SumI2OutMin=[]  SumI2OutMax=[]  SumI3OutMin=[]  SumI3OutMax=[]  SumDOutMin=[]  SumDOutMax=[]  SaturationOutMin=[]  SaturationOutMax=[]  IntegratorContinuousStateAttributes=''  IntegratorStateMustResolveToSignalObject=off  IntegratorRTWStateStorageClass=Auto  FilterContinuousStateAttributes=''  FilterStateMustResolveToSignalObject=off  FilterRTWStateStorageClass=Auto  DifferentiatorICPrevScaledInput=0  DifferentiatorOutMin=[]  DifferentiatorOutMax=[]
  az Response : Scope
  "e Az " : Scope
  q Gain : Gain  Gain=Kq
  del_e : Outport
  wires:
  az Control/1 -> Sum1/1
  Sum1/1 -> Discrete-Time Integrator/1
  Sum/1 -> "e Az "/1, az Control/1
  KP/1 -> Sum10/1
  Sum10/1 -> KI/1
  KI/1 -> Discrete-Time Integrator2/1
  Discrete-Time Integrator2/1 -> Sum5/1
  Demux1/3 -> Sum1/2, Sum5/2, Sum10/2  "q"
  Sum5/1 -> KG/1
  Sum9/1 -> KP/1
  Discrete-Time Integrator/1 -> q Gain/1
  q Gain/1 -> del_e/1
  Demux1/1 -> Sum/1, Sum9/2, Mux/1  "Az ref"
  Demux1/2 -> Sum/2, Mux/2, Sum9/1  "Az"
  Mux/1 -> az Response/1
  Switch Condition/1 -> Switch del_e/2
  Zero/1 -> Switch del_e/3
  In/1 -> Switch del_e/1
  Switch del_e/1 -> Demux1/1

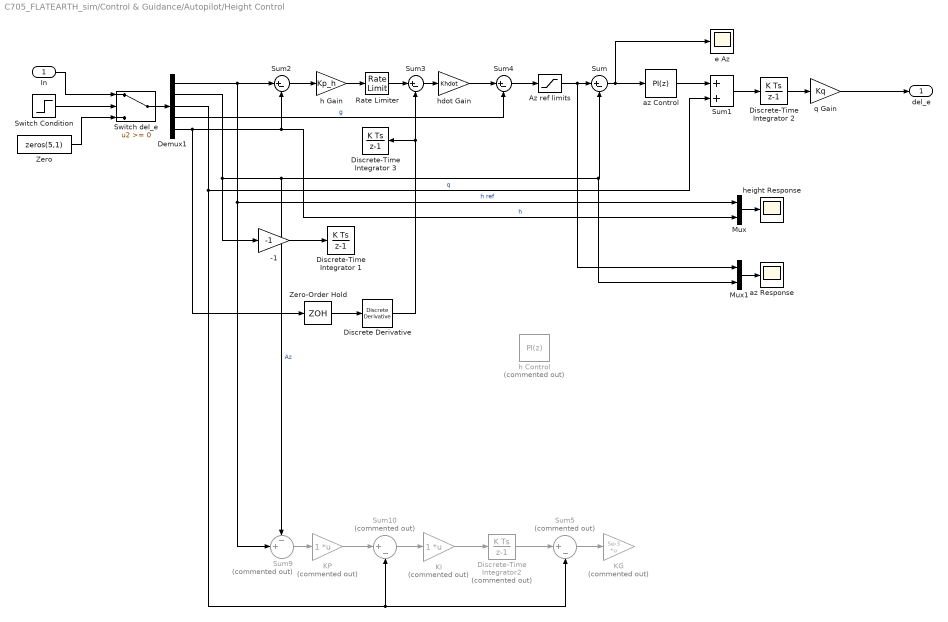
== system C705_FLATEARTH_sim/Control & Guidance/Autopilot/Height Control ==
  In : Inport
  -1 : Gain  Gain=-1
  Az ref limits : Saturate  UpperLimit=20  LowerLimit=-20
  Demux1 : Demux  Outputs=5
  Discrete Derivative : simulink/Discrete/Discrete Derivative  gainval=1.0  ICPrevScaledInput=0.0  OutMin=[]  OutMax=[]  OutDataType=fixdt(1, 16)  OutScaling=2^-10  DoSatur=off
  Discrete-Time Integrator 1 : DiscreteIntegrator  InitialConditionSetting=State (most efficient)  SampleTime=Ts_ap  ICPrevOutput=DiscIntNeverNeededParam  ICPrevScaledInput=DiscIntNeverNeededParam
  Discrete-Time Integrator 2 : DiscreteIntegrator  InitialConditionSetting=State (most efficient)  SampleTime=Ts_ap  ICPrevOutput=DiscIntNeverNeededParam  ICPrevScaledInput=DiscIntNeverNeededParam
  Discrete-Time Integrator 3 : DiscreteIntegrator  InitialConditionSetting=State (most efficient)  SampleTime=Ts_ap  ICPrevOutput=DiscIntNeverNeededParam  ICPrevScaledInput=DiscIntNeverNeededParam
  Discrete-Time Integrator2 : DiscreteIntegrator  Commented=on  SampleTime=Ts_ap  ICPrevOutput=DiscIntNeverNeededParam  ICPrevScaledInput=DiscIntNeverNeededParam
  KG : Gain  Commented=on  Gain=5e-3  Multiplication=Matrix(K*u)  SaturateOnIntegerOverflow=on  OutDataTypeStr=Inherit: Same as input  ParamDataTypeStr=Inherit: Same as input
  KI : Gain  Commented=on  Multiplication=Matrix(K*u)  SaturateOnIntegerOverflow=on  OutDataTypeStr=Inherit: Same as input  ParamDataTypeStr=Inherit: Same as input
  KP : Gain  Commented=on  Multiplication=Matrix(K*u)  SaturateOnIntegerOverflow=on  OutDataTypeStr=Inherit: Same as input  ParamDataTypeStr=Inherit: Same as input
  Mux : Mux  Inputs=2
  Mux1 : Mux  Inputs=2
  Rate Limiter : RateLimiter  RisingSlewLimit=20  FallingSlewLimit=-20  SampleTimeMode=inherited
  Sum{,2..4} (4 alike) : Sum  Inputs=|+-  SaturateOnIntegerOverflow=on
  Sum1 : Sum  SaturateOnIntegerOverflow=on
  Sum10 : Sum  Commented=on  Inputs=|+-  SaturateOnIntegerOverflow=on  InputSameDT=on  OutDataTypeStr=Inherit: Same as first input
  Sum5 : Sum  Commented=on  Inputs=|+-  SaturateOnIntegerOverflow=on  InputSameDT=on  OutDataTypeStr=Inherit: Same as first input
  Sum9 : Sum  Commented=on  Inputs=-+|  SaturateOnIntegerOverflow=on  InputSameDT=on  OutDataTypeStr=Inherit: Same as first input
  Switch Condition : Step  Time=t_activate_del_e  Before=-1  SampleTime=0
  Switch del_e : Switch
  Zero : Constant  Value=zeros(5,1)  SampleTime=Ts_guid
  Zero-Order Hold : ZeroOrderHold  SampleTime=Ts_ap
  az Control : simulink/Continuous/PID Controller  Controller=PI  TimeDomain=Discrete-time  SampleTime=Ts_ap  IntegratorMethod=Trapezoidal  FilterMethod=Forward Euler  Form=Parallel  UseFilter=on  ControllerParametersSource=internal  P=Kp_az  I=Ki_az  D=0  N=12  InitialConditionSource=internal  InitialConditionForIntegrator=0  InitialConditionForFilter=0  ExternalReset=none  LimitOutput=off  UpperSaturationLimit=inf  LowerSaturationLimit=-inf  LinearizeAsGain=off  AntiWindupMode=none  Kb=1  TrackingMode=off  Kt=1  PParamMin=[]  PParamMax=[]  IParamMin=[]  IParamMax=[]  DParamMin=[]  DParamMax=[]  NParamMin=[]  NParamMax=[]  KbParamMin=[]  KbParamMax=[]  KtParamMin=[]  KtParamMax=[]  POutMin=[]  POutMax=[]  IOutMin=[]  IOutMax=[]  DOutMin=[]  DOutMax=[]  NOutMin=[]  NOutMax=[]  KbOutMin=[]  KbOutMax=[]  KtOutMin=[]  KtOutMax=[]  IntegratorOutMin=[]  IntegratorOutMax=[]  FilterOutMin=[]  FilterOutMax=[]  SumOutMin=[]  SumOutMax=[]  SumI1OutMin=[]  SumI1OutMax=[]  SumI2OutMin=[]  SumI2OutMax=[]  SumI3OutMin=[]  SumI3OutMax=[]  SumDOutMin=[]  SumDOutMax=[]  SaturationOutMin=[]  SaturationOutMax=[]  IntegratorContinuousStateAttributes=''  IntegratorStateMustResolveToSignalObject=off  IntegratorRTWStateStorageClass=Auto  FilterContinuousStateAttributes=''  FilterStateMustResolveToSignalObject=off  FilterRTWStateStorageClass=Auto  DifferentiatorICPrevScaledInput=0  DifferentiatorOutMin=[]  DifferentiatorOutMax=[]
  az Response : Scope
  "e Az " : Scope
  h Control : simulink/Continuous/PID Controller  Commented=on  Controller=PI  TimeDomain=Discrete-time  SampleTime=Ts_ap  IntegratorMethod=Trapezoidal  FilterMethod=Forward Euler  Form=Parallel  UseFilter=on  ControllerParametersSource=internal  P=Kp_h  I=Ki_h  D=0  N=12  InitialConditionSource=internal  InitialConditionForIntegrator=0  InitialConditionForFilter=0  ExternalReset=none  LimitOutput=off  UpperSaturationLimit=inf  LowerSaturationLimit=-inf  LinearizeAsGain=off  AntiWindupMode=none  Kb=1  TrackingMode=off  Kt=1  PParamMin=[]  PParamMax=[]  IParamMin=[]  IParamMax=[]  DParamMin=[]  DParamMax=[]  NParamMin=[]  NParamMax=[]  KbParamMin=[]  KbParamMax=[]  KtParamMin=[]  KtParamMax=[]  POutMin=[]  POutMax=[]  IOutMin=[]  IOutMax=[]  DOutMin=[]  DOutMax=[]  NOutMin=[]  NOutMax=[]  KbOutMin=[]  KbOutMax=[]  KtOutMin=[]  KtOutMax=[]  IntegratorOutMin=[]  IntegratorOutMax=[]  FilterOutMin=[]  FilterOutMax=[]  SumOutMin=[]  SumOutMax=[]  SumI1OutMin=[]  SumI1OutMax=[]  SumI2OutMin=[]  SumI2OutMax=[]  SumI3OutMin=[]  SumI3OutMax=[]  SumDOutMin=[]  SumDOutMax=[]  SaturationOutMin=[]  SaturationOutMax=[]  IntegratorContinuousStateAttributes=''  IntegratorStateMustResolveToSignalObject=off  IntegratorRTWStateStorageClass=Auto  FilterContinuousStateAttributes=''  FilterStateMustResolveToSignalObject=off  FilterRTWStateStorageClass=Auto  DifferentiatorICPrevScaledInput=0  DifferentiatorOutMin=[]  DifferentiatorOutMax=[]
  h Gain : Gain  Gain=Kp_h
  hdot Gain : Gain  Gain=Khdot
  height Response : Scope
  q Gain : Gain  Gain=Kq
  del_e : Outport
  wires:
  az Control/1 -> Sum1/1
  Sum1/1 -> Discrete-Time Integrator 2/1
  Sum/1 -> "e Az "/1, az Control/1
  KP/1 -> Sum10/1
  Sum10/1 -> KI/1
  KI/1 -> Discrete-Time Integrator2/1
  Discrete-Time Integrator2/1 -> Sum5/1
  Demux1/3 -> Sum1/2, Sum5/2, Sum10/2  "q"
  Sum5/1 -> KG/1
  Sum9/1 -> KP/1
  Discrete-Time Integrator 2/1 -> q Gain/1
  q Gain/1 -> del_e/1
  Demux1/1 -> Sum9/2, Mux/1, Sum2/1  "h ref"
  Demux1/2 -> -1/1, Sum9/1, Mux1/2, Sum/2  "Az"
  Mux/1 -> height Response/1
  Switch Condition/1 -> Switch del_e/2
  Zero/1 -> Switch del_e/3
  In/1 -> Switch del_e/1
  Switch del_e/1 -> Demux1/1
  Sum2/1 -> h Gain/1
  h Gain/1 -> Rate Limiter/1
  Rate Limiter/1 -> Sum3/1
  Discrete Derivative/1 -> Discrete-Time Integrator 3/1, Sum3/2
  Sum3/1 -> hdot Gain/1
  hdot Gain/1 -> Sum4/1
  Demux1/4 -> Sum4/2  "g"
  Mux1/1 -> az Response/1
  -1/1 -> Discrete-Time Integrator 1/1
  Az ref limits/1 -> Mux1/1, Sum/1
  Demux1/5 -> Zero-Order Hold/1, Mux/2, Sum2/2  "h"
  Zero-Order Hold/1 -> Discrete Derivative/1
  Sum4/1 -> Az ref limits/1
